simulink model "oe_ex1"  (Simulink 5.0)
settings: Solver=ode45  StartTime=0.0  StopTime=10.0  RelTol=1e-3
settings Model: Creator=kannan  LastModifiedBy=kannan  ExtModeAutoUpdateStatusClock=off

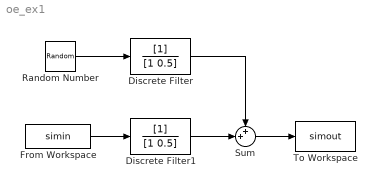
== system oe_ex1 ==
  Discrete Filter : DiscreteFilter  Denominator=[1 0.5]
  Discrete Filter1 : DiscreteFilter  Denominator=[1 0.5]
  From Workspace : FromWorkspace  VariableName=simin  SampleTime=0
  Random Number : RandomNumber  SampleTime=0
  Sum : Sum  Inputs=++|  SaturateOnIntegerOverflow=on
  To Workspace : ToWorkspace  VariableName=simout  SampleTime=-1  SaveFormat=Structure
  wires:
  Random Number/1 -> Discrete Filter/1
  From Workspace/1 -> Discrete Filter1/1
  Discrete Filter/1 -> Sum/1
  Discrete Filter1/1 -> Sum/2
  Sum/1 -> To Workspace/1
